simulink model "vj7"  (R2020b)
settings: Solver=VariableStepAuto  StartTime=0.0  StopTime=10.0  RelTol=1e-3
values from neighbouring files (symbols this model uses):
  g = 9.81    [vj7.m]
  I = M*L^2/12    (= 0.0238203375)    [vj7.m]
  J = 2/5*m*r^2    (= 1.08e-05)    [vj7.m]
  K = lqr(A, B, Q, R)    [vj7.m]
  m = 0.12    [vj7.m]
  r = 0.015    [vj7.m]
settings Model: Creator=dominik  LastModifiedBy=dominik

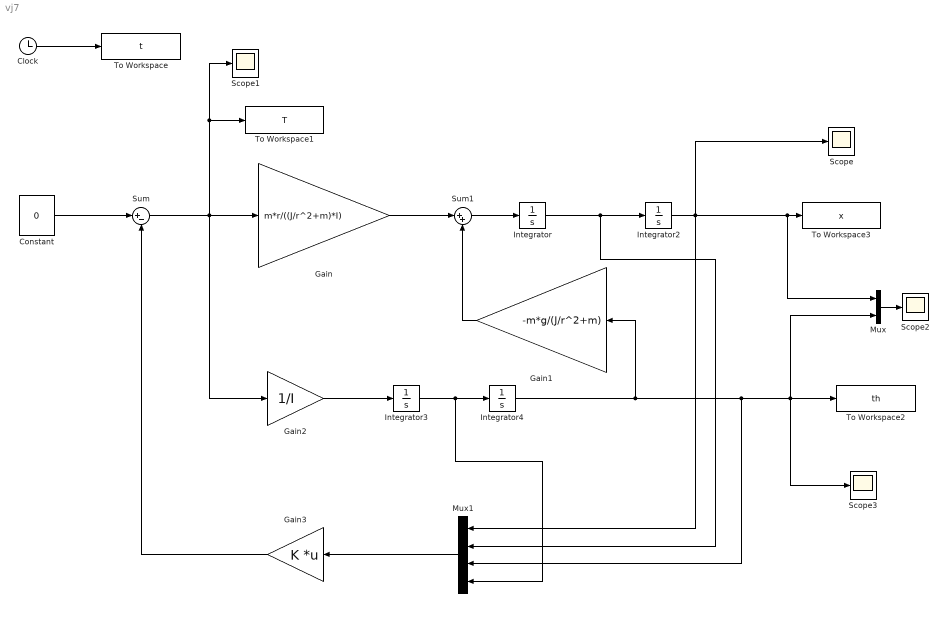
== system vj7 ==
  Clock : Clock
  Constant : Constant  Value=0
  Gain : Gain  Gain=m*r/((J/r^2+m)*I)
  Gain1 : Gain  Gain=-m*g/(J/r^2+m)
  Gain2 : Gain  Gain=1/I
  Gain3 : Gain  Gain=K  Multiplication=Matrix(K*u)
  Integrator : Integrator
  Integrator2 : Integrator  InitialCondition=0.1
  Integrator3 : Integrator
  Integrator4 : Integrator
  Mux : Mux  Inputs=2
  Mux1 : Mux
  Scope{,1..3} (4 alike) : Scope
  Sum : Sum  Inputs=|+-
  Sum1 : Sum  Inputs=|++
  To Workspace : ToWorkspace  VariableName=t  SaveFormat=Timeseries  SampleTime=-1
  To Workspace1 : ToWorkspace  VariableName=T  SaveFormat=Timeseries  SampleTime=-1
  To Workspace2 : ToWorkspace  VariableName=th  SaveFormat=Timeseries  SampleTime=-1
  To Workspace3 : ToWorkspace  VariableName=x  SaveFormat=Timeseries  SampleTime=-1
  wires:
  Constant/1 -> Sum/1
  Sum/1 -> Scope1/1, To Workspace1/1, Gain2/1, Gain/1
  Gain/1 -> Sum1/1
  Gain1/1 -> Sum1/2
  Sum1/1 -> Integrator/1
  Gain2/1 -> Integrator3/1
  Mux1/1 -> Gain3/1
  Gain3/1 -> Sum/2
  Integrator4/1 -> Gain1/1, Mux1/3, Scope3/1, Mux/2, To Workspace2/1
  Integrator2/1 -> Mux1/1, Scope/1, Mux/1, To Workspace3/1
  Mux/1 -> Scope2/1
  Integrator3/1 -> Mux1/4, Integrator4/1
  Integrator/1 -> Mux1/2, Integrator2/1
  Clock/1 -> To Workspace/1
